simulink model "mDisableBusWithVardim"
settings: Solver=FixedStepDiscrete  StartTime=0.0  StopTime=10  RelTol=1e-3
PreLoadFcn:
  | load hvar_dims_etvs_itvs_bus3.mat
CloseFcn:
  | %evalin('base', 'clear TopBus MidBus BottomBus');
settings Model: Creator=sjha  LastModifiedBy=hungdang
settings DataIOCC: LimitDataPoints=on  SaveFormat=StructureWithTime  SignalLoggingSaveFormat=ModelDataLogs  ReturnWorkspaceOutputs=off  StateSaveName=x  OutputSaveName=y
settings OptimizationCC: InlineParams=on  ExpressionDepthLimit=2147483647  InitFltsAndDblsToZero=on  EfficientMapNaN2IntZero=off  LifeSpan=inf  SimCompilerOptimization=Off
settings DebuggingCC: UnderspecifiedInitializationDetection=Classic  MergeDetectMultiDrivingBlocksExec=none  SolverPrmCheckMsg=warning  FcnCallInpInsideContextMsg=UseLocalSettings  FrameProcessingCompatibilityMsg=warning  StateNameClashWarn=warning  StrictBusMsg=ErrorOnBusTreatedAsVector  SFUnexpectedBacktrackingDiag=warning  SFNoUnconditionalDefaultTransitionDiag=warning
settings HardwareCC: ProdBitPerPointer=32  ProdLargestAtomicFloat=None  ProdIntDivRoundTo=Undefined  ProdEndianess=Unspecified  ProdWordSize=32  ProdHWDeviceType=32-bit Generic
settings ModelReferenceCC: PropagateVarSize=During execution  PropagateSignalLabelsOutOfModel=off
settings SFSimCC: SimUseLocalCustomCode=off
settings RTWCC: GenerateReport=on  RetainRTWFile=on  RTWUseLocalCustomCode=off  LaunchReport=on  TargetLang=C++  RTWCompilerOptimization=Off
settings CodeAppCC: MaxIdLength=127  CustomSymbolStrType=$N$R$M
settings GRTTargetCC: CodeReplacementLibrary=ANSI_C  GeneratePreprocessorConditionals=Disable all  CombineOutputUpdateFcns=off  CPPClassGenCompliant=off  GRTInterface=on

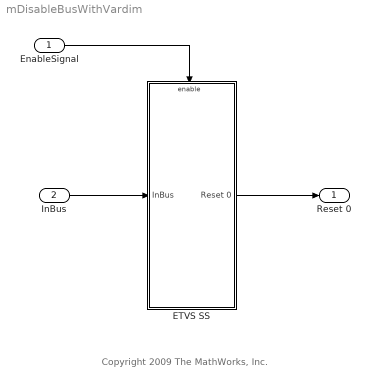
== system mDisableBusWithVardim ==
  note: Copyright 2009 The MathWorks, Inc.
  EnableSignal : Inport
  InBus : Inport  Port=2  OutDataTypeStr=Bus: TopBus  Interpolate=off  BusOutputAsStruct=on
  ETVS SS : Subsystem  TreatAsAtomicUnit=on
  Reset 0 : Outport  OutDataTypeStr=Bus: TopBus  OutputWhenDisabled=reset  InitialOutput=0
  wires:
  InBus/1 -> ETVS SS/1(InBus)
  ETVS SS/1(Reset 0) -> Reset 0/1
  EnableSignal/1 -> ETVS SS/Enable

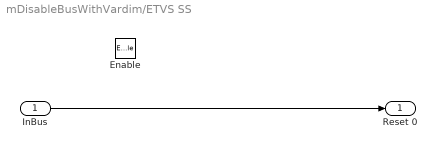
== system mDisableBusWithVardim/ETVS SS ==
  InBus : Inport
  Enable : EnablePort  StatesWhenEnabling=reset  PropagateVarSize=During execution
      settings: AttributesFormatString=%<PropagateVarSize>
  Reset 0 : Outport  OutputWhenDisabled=reset  InitialOutput=0
  wires:
  InBus/1 -> Reset 0/1
